simulink library "alfa_wall_in"  (R2018b)
settings: Solver=ode45  StartTime=0.0  StopTime=10.0  RelTol=1e-3  EnableMultiTasking=on
settings Model: Creator=lena.frank  LastModifiedBy=drhf
settings DataIOCC: LimitDataPoints=on  SaveFormat=Array  SignalLoggingSaveFormat=ModelDataLogs
settings OptimizationCC: ExpressionDepthLimit=2147483647  LifeSpan=inf
settings DebuggingCC: UnderspecifiedInitializationDetection=Classic  MergeDetectMultiDrivingBlocksExec=none  SolverPrmCheckMsg=warning  FcnCallInpInsideContextMsg=warning  StateNameClashWarn=warning  SFUnexpectedBacktrackingDiag=warning  SFNoUnconditionalDefaultTransitionDiag=warning  SFExecutionAtInitializationDiag=none
settings HardwareCC: ProdBitPerPointer=32  ProdBitPerSizeT=32  ProdBitPerPtrDiffT=32  ProdLargestAtomicFloat=None  ProdIntDivRoundTo=Undefined  ProdEndianess=Unspecified  ProdWordSize=32  ProdHWDeviceType=32-bit Generic
settings ModelReferenceCC: PropagateSignalLabelsOutOfModel=off
settings SFSimCC: SimUseLocalCustomCode=off
settings RTWCC: RTWUseLocalCustomCode=off
settings CodeAppCC: StateflowObjectComments=on
settings GRTTargetCC: TargetLangStandard=C89/C90 (ANSI)  GeneratePreprocessorConditionals=Disable all  CombineOutputUpdateFcns=off  GRTInterface=on
settings ConfigComp: CovMetricSettings=dw  CovHtmlReporting=on  CovSaveCumulativeToWorkspaceVar=on  CovSaveSingleToWorkspaceVar=on  CovExternalEMLEnable=off

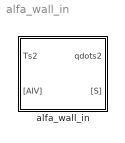
== system alfa_wall_in ==
  alfa_wall_in : Subsystem  mask(ALFA){active=0, emission_in=0.7, wallsurface=1}
      mask prompts: active "Active layer (0 / 1)"; emission_in "Longwave emissivity of surface (0..1)"; wallsurface "Wall surface in m²"
      mask help:
      | Convective and radiative heat transfer at the INDOOR SURFACE of a VERTICAL OUTER WALL.
      |
      | [AIV] : conditions of zone node,
      | Ts : temperature of wall surface, °C,
      | qdots : specific heat flow into wall construction, W/m^2,
      | [S] : heat and air flow to zone node.
      mask Help: web(fullfile(path_carnot('help'),'alfa_wall_in.html'),'-helpbrowser')

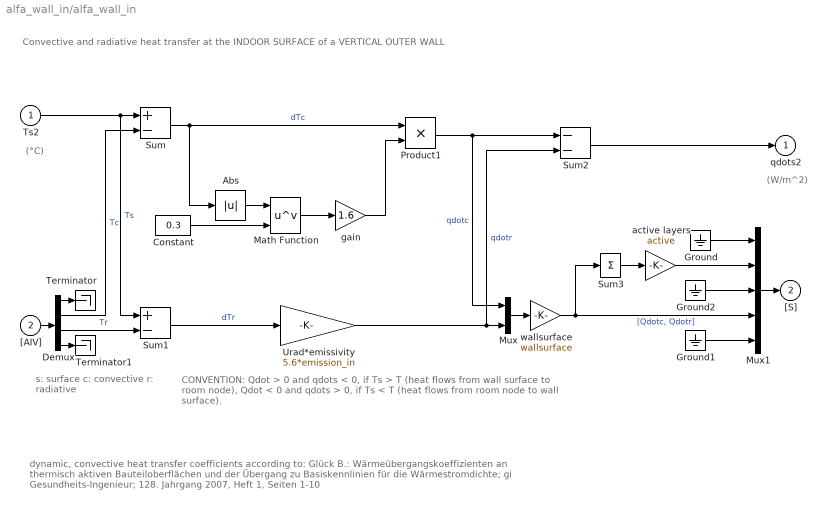
== system alfa_wall_in/alfa_wall_in ==
  note: dynamic, convective heat transfer coefficients according to: Glück B.: Wärmeübergangskoeffizienten an thermisch aktiven Bauteiloberflächen
      | und der Übergang zu Basiskennlinien für die Wärmestromdichte; gi Gesundheits-Ingenieur; 128. Jahrgang 2007, Heft 1, Seiten 1-10
  note: s: surface
      | c: convective
      | r: radiative
  note: CONVENTION:
      | Qdot > 0 and qdots < 0, if Ts > T (heat flows from wall surface to room node),
      | Qdot < 0 and qdots > 0, if Ts < T (heat flows from room node to wall surface).
  note: Convective and radiative heat transfer at the INDOOR SURFACE of a VERTICAL OUTER WALL
  note: (W/m^2)
  note: (°C)
  Ts2 : Inport
  "[AIV]" : Inport  Port=2
  Abs : Abs
  Constant : Constant  Value=0.3
  Demux : Demux  Outputs=[1 1 1 6]
  Ground : Ground
  Ground1 : Ground
  Ground2 : Ground
  Math Function : Math  Operator=pow  SaturateOnIntegerOverflow=on
  Mux : Mux  Inputs=2
  Mux1 : Mux  Inputs=[4 1 1 2 5]
  Product1 : Product  SaturateOnIntegerOverflow=on  RndMeth=Zero  InputSameDT=on  OutDataTypeStr=Inherit: Same as first input
  Sum : Sum  Inputs=+-  SaturateOnIntegerOverflow=on  InputSameDT=on  OutDataTypeStr=Inherit: Same as first input
  Sum1 : Sum  Inputs=+-  SaturateOnIntegerOverflow=on  InputSameDT=on  OutDataTypeStr=Inherit: Same as first input
  Sum2 : Sum  Inputs=--  SaturateOnIntegerOverflow=on  InputSameDT=on  OutDataTypeStr=Inherit: Same as first input
  Sum3 : Sum  Inputs=1  SaturateOnIntegerOverflow=on  InputSameDT=on  OutDataTypeStr=Inherit: Same as first input
  Terminator : Terminator
  Terminator1 : Terminator
  Urad*emissivity : Gain  Gain=5.6*emission_in  SaturateOnIntegerOverflow=on  OutDataTypeStr=Inherit: Same as input  ParamDataTypeStr=Inherit: Same as input
  active layers : Gain  Gain=active  SaturateOnIntegerOverflow=on  OutDataTypeStr=Inherit: Same as input  ParamDataTypeStr=Inherit: Same as input
  gain : Gain  Gain=1.6  SaturateOnIntegerOverflow=on  OutDataTypeStr=Inherit: Same as input  ParamDataTypeStr=Inherit: Same as input
  wallsurface : Gain  Gain=wallsurface  SaturateOnIntegerOverflow=on  OutDataTypeStr=Inherit: Same as input  ParamDataTypeStr=Inherit: Same as input
  qdots2 : Outport
  "[S]" : Outport  Port=2
  wires:
  gain/1 -> Product1/2
  Math Function/1 -> gain/1
  Abs/1 -> Math Function/1
  Constant/1 -> Math Function/2
  Sum/1 -> Abs/1, Product1/1  "dTc"
  Product1/1 -> Mux/1, Sum2/1  "qdotc"
  Demux/3 -> Sum1/2  "Tr"
  Ts2/1 -> Sum1/1, Sum/1  "Ts"
  Mux/1 -> wallsurface/1
  Urad*emissivity/1 -> Sum2/2, Mux/2  "qdotr"
  Sum1/1 -> Urad*emissivity/1  "dTr"
  Demux/2 -> Sum/2  "Tc"
  Demux/1 -> Terminator/1
  "[AIV]"/1 -> Demux/1
  Demux/4 -> Terminator1/1
  Sum2/1 -> qdots2/1
  wallsurface/1 -> Mux1/4, Sum3/1  "[Qdotc, Qdotr]"
  Sum3/1 -> active layers/1
  Ground/1 -> Mux1/1
  Ground1/1 -> Mux1/5
  Mux1/1 -> "[S]"/1
  Ground2/1 -> Mux1/3
  active layers/1 -> Mux1/2
